simulink model "stanleyHighway"  (R2020b)
settings: Solver=VariableStepAuto  StartTime=0.0  StopTime=50  FixedStep=0.001  RelTol=1e-3
PreLoadFcn:
  | velocityProfile
  | setUpModel
  | close
model workspace (MAT data in the model file):
  firstWarning = 0
  originalScenarioChecksum = 'F73A6DA3C723D3CA73A6F931B7A52A9C'
undefined symbols (not defined in the file or in its folder): curvature, direction, dislt, distancecovered, gradbp, psi_o, q11, thetaRefab, velt_res, X_o, xRef2s, Y_o, yRef2s
libraries: vehdynlibtirecommon x4, autolibutils x4, simulink_extras x3, simulink x3, drivingvehiclecontroller x2, vehdynlibviscommon x1, drivingscenarioandsensors x1, vehdynlibtire x1, sim3dlib x1, vdynlib x1, autolibshared x1
settings Model: PacingRate=0.700000  Creator=valakshe  LastModifiedBy=valakshe

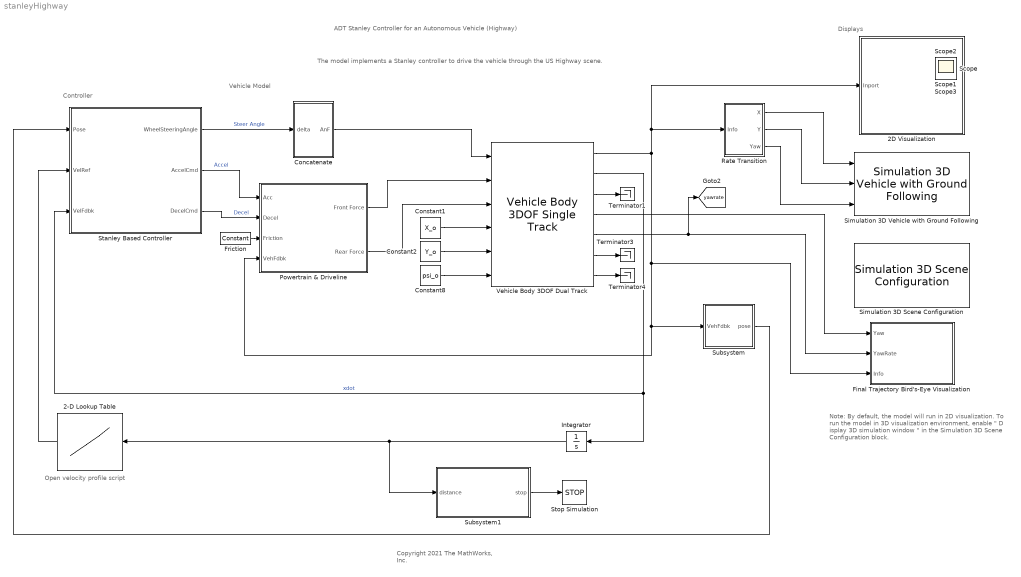
== system stanleyHighway ==
  note: Open velocity profile script
  note: Note: By default, the model will run in 2D visualization. To run the model in 3D visualization
      | environment, enable " D isplay 3D simulation window " in the Simulation 3D Scene Configuration block.
  note: Copyright 2021 The MathWorks, Inc.
  note: Controller
  note: Vehicle Model
  note: ADT Stanley Controller for an Autonomous Vehicle
      | (Highway)
  note: Displays
  note: The model implements a Stanley controller to drive the vehicle through the US Highway scene.
  2-D Lookup Table : Lookup_n-D  NumberOfTableDimensions=1  BreakpointsForDimension1=dislt;  BreakpointsForDimension2=q11(:,2)  Table=velt_res;  InterpMethod=Cubic spline  InternalRulePriority=Speed  RndMeth=Simplest  InputSameDT=on
  2D Visualization : Subsystem
      mask Display: image("visualization.JPG");
  Concatenate : Subsystem
  Constant1 : Constant  Value=X_o
  Constant2 : Constant  Value=Y_o
  Constant8 : Constant  Value=psi_o
  Final Trajectory Bird's-Eye Visualization : Subsystem
  Friction : vehdynlibtirecommon/Constant  const=1  numWheels=4
      settings: SourceProductBaseCode=VE
  Integrator : Integrator  InitialCondition=sqrt((X_o).^2+(Y_o).^2)
  Powertrain & Driveline : Subsystem
      mask Display: image('vdbslibpt.png');
  Rate Transition : Subsystem
  Simulation 3D Scene Configuration : sim3dlib/Simulation 3D Scene Configuration  Priority=1  ProjectFormat=Default Scenes  SceneDesc=US highway  ProjectName=C:\Fdrive\UnrealAutonomousVehicle\8MileUnrealexe\AutoVrtlEnv.exe  ScenePath=8mile  UEProjPath=C:\Local\AutoVrtlEnv\AutoVrtlEnv.uproject  vehTagList={'Scene Origin';'SimulinkVehicle1'}  vehTag=SimulinkVehicle1  OpVisEn=off  Ts=.05  EnableWindow=on  sensorTag=MainCamera1  sensorId=1  sensorName=MainCamera1  mountLoc=Origin  offsetFlag=off  tmountOffset=[0, 0, 0]  rmountOffset=[0, 0, 0]  HorizontalResolution=1280  VerticalResolution=720  HorizontalFOV=60  mountPoint=[0 0 0]  mountOrientation=[0 0 0]  aMode=2  ID=1
      settings: SourceProductBaseCode=DR,UV,VE
  Simulation 3D Vehicle with Ground Following : vdynlib/Vehicle Scenarios/Sim3D/Sim3D Vehicle/Components/Simulation 3D Vehicle with Ground Following  Priority=-1  PassVehMesh=Hatchback  VehColor=Green  InitialPos=[X_o,Y_o,-1]  InitialRot=[0, 0, psi_o]  ActorName=SimulinkVehicle1  SampleTime=-1  ActorType=SimulinkVehicle  ID=1  aMode=2  ActorTag=SimulinkVehicle1  CoordinateScheme=SAE
      settings: SourceProductBaseCode=VE
  Stanley Based Controller : Subsystem  VariantControl=Stanley
  Stop Simulation : Stop
  Subsystem : Subsystem
  Subsystem1 : Subsystem
  Terminator1 : Terminator
  Terminator3 : Terminator
  Terminator4 : Terminator
  Vehicle Body 3DOF Dual Track : autolibshared/Vehicle Body 3DOF Single Track  trackMode=Dual  inputMode=External forces  frontSteerMode=on  rearSteerMode=off  windMode=off  muMode=off  extFMode=off  extMMode=off  htchFMode=off  htchMMode=off  extXo=on  extpsio=on  extxdoto=off  extro=off  extYo=on  extTamb=off  extydoto=off  aMode=2  NF=2  NR=2  m=2000  a=1.4  b=1.6  h=0.35  dh=1  hh=0.2  X_o=0  xdot_o=velt_res(1)  CalphaMode=off  sigmaMode=on  d=0  hl=0  w=[1.4,1.4]  Cy_f=12e3  Cy_r=11e3  sigma_f=.1  sigma_r=.1  alpha_f_brk=[-.1 .1]  Cy_f_data=[-9e3 9e3]  alpha_r_brk=[-.1 .1]  Cy_r_data=[-9e3 9e3]  Y_o=0  ydot_o=0  Izz=4000  psi_o=0  r_o=0  Af=2  Cd=.3  Cl=.1  Cpm=.1  beta_w=[0:0.01:0.3]  Cs=[0:0.03:0.9]  Cym=[0:0.01:0.3]  Pabs=101325  Tair=273  g=9.81  mu=1  xdot_tol=.01  Fznom=5000  Fxtire_sat=7e4  Fytire_sat=7e4  longOff=0  latOff=0  vertOff=0  wrapAng=off
      settings: SourceProductBaseCode=PW,MT,UV,VE,VP
  Scope{,1..3} (4 alike) : Scope
  tag scope: yawrate=global
  wires:
  Vehicle Body 3DOF Dual Track/7 -> Terminator4/1
  Vehicle Body 3DOF Dual Track/4 -> Final Trajectory Bird's-Eye Visualization/1(Yaw)
  Powertrain & Driveline/1(Front Force) -> Vehicle Body 3DOF Dual Track/2
  Stanley Based Controller/3(DecelCmd) -> Powertrain & Driveline/2(Decel)  "Decel"
  Vehicle Body 3DOF Dual Track/1 -> Subsystem/1(VehFdbk), Powertrain & Driveline/4(VehFdbk), Final Trajectory Bird's-Eye Visualization/3(Info), Rate Transition/1(Info), 2D Visualization/1(Inport)
  Constant1/1 -> Vehicle Body 3DOF Dual Track/4
  Stanley Based Controller/1(WheelSteeringAngle) -> Concatenate/1(delta)  "Steer Angle"
  Vehicle Body 3DOF Dual Track/2 -> Integrator/1, Stanley Based Controller/3(VelFdbk)  "xdot"
  Vehicle Body 3DOF Dual Track/3 -> Terminator1/1
  Concatenate/1(AnF) -> Vehicle Body 3DOF Dual Track/1
  Vehicle Body 3DOF Dual Track/6 -> Terminator3/1
  Constant8/1 -> Vehicle Body 3DOF Dual Track/6
  Rate Transition/1(X) -> Simulation 3D Vehicle with Ground Following/1
  Powertrain & Driveline/2(Rear Force) -> Vehicle Body 3DOF Dual Track/3
  Vehicle Body 3DOF Dual Track/5 -> Final Trajectory Bird's-Eye Visualization/2(YawRate), [yawrate]
  Rate Transition/3(Yaw) -> Simulation 3D Vehicle with Ground Following/3
  Rate Transition/2(Y) -> Simulation 3D Vehicle with Ground Following/2
  Stanley Based Controller/2(AccelCmd) -> Powertrain & Driveline/1(Acc)  "Accel"
  Constant2/1 -> Vehicle Body 3DOF Dual Track/5
  Friction/1 -> Powertrain & Driveline/3(Friction)
  Subsystem/1(pose) -> Stanley Based Controller/1(Pose)
  Subsystem1/1(stop) -> Stop Simulation/1
  2-D Lookup Table/1 -> Stanley Based Controller/2(VelRef)
  Integrator/1 -> Subsystem1/1(distance), 2-D Lookup Table/1

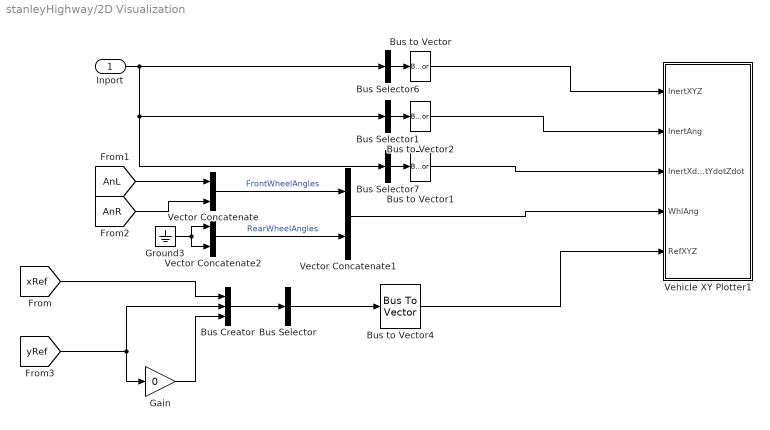
== system stanleyHighway/2D Visualization ==
  Inport : Inport
  Bus Creator : BusCreator  Inputs=3
  Bus Selector : BusSelector  OutputSignals=signal1,signal2,signal3  OutputAsBus=on
  Bus Selector1 : BusSelector  OutputSignals=InertFrm.Cg.Ang.phi,InertFrm.Cg.Ang.theta,InertFrm.Cg.Ang.psi  OutputAsBus=on
  Bus Selector6 : BusSelector  OutputSignals=InertFrm.Geom.Disp.X,InertFrm.Geom.Disp.Y,InertFrm.Geom.Disp.Z  OutputAsBus=on
  Bus Selector7 : BusSelector  OutputSignals=InertFrm.Geom.Vel.Xdot,InertFrm.Geom.Vel.Ydot,InertFrm.Geom.Vel.Zdot  OutputAsBus=on
  Bus to Vector{,1..2,4} (4 alike) : BusToVector
  Gain : Gain  Gain=0
  Ground3 : Ground
  Vector Concatenate : Concatenate
  Vector Concatenate1 : Concatenate
  Vector Concatenate2 : Concatenate
  Vehicle XY Plotter1 : Subsystem  mask(Vehicle XY Plotter){extRef=on, extStats=off, extTireF=off, a=2, b=2, w=2, figBorder=10, bufferSize=1024, velNorm=5, tireFNorm=1000, pltDT=0.2}
      mask prompts: extRef "Plot path reference, extRef"; extStats "Display speed, RPM and Gear"; extTireF "Display tire forces"; a "Distance to front axle from CG, a [m]:"; b "Distance to rear axle from CG, b [m]:"; w "Track width, w [m]:"; figBorder "Distance to figure borders, figBorder [m]:"; bufferSize "Path buffer sampe size, bufferSize []:"; velNorm "Velocity vector scaling, velNorm [m*s/m]:"; tireFNorm "Tire force vector scaling, tireFNorm [m/N]:"; pltDT "Plot update rate, pltDT [s]:"
      mask help:
      | This block will display a MATLAB figure which indicates the vehicle path, current position and heading velocity.
      | An optional path reference is also provided.
      mask init:
      | block = gcb;
      | if autoblkschecksimstopped(block)
      |     ParamNames = {'extRef';'extStats';'extTireF';'extTireF'};
      |     PortNames = {'RefXYZ';'Stats';'TireFx';'TireFy'};
      |     for idx=1:length(PortNames)
      |         InportOption  = {'built-in/Ground', [PortNames{idx}, ' Ground'];...
      |             'built-in/Inport',PortNames{idx}};
      |         if ~strcmp(get_param(block,ParamNames{idx}),'on')
      |             NewBlkHdl = autoblksreplaceblock(block, InportOption, 1);
      |             set_param(NewBlkHdl, 'ShowName', 'off');
      |         else
      |             autoblksreplaceblock(block, InportOption, 2);
      |         end
      |     end
      |     InportNames = {'InertXYZ';'InertAng';'InertXdotYdotZdot';'WhlAng';'RefXYZ';'Stats';'TireFx';'TireFy'};
      |     FoundNames = get_param(find_system(block, 'LookUnderMasks', 'all', 'SearchDepth', 1, 'FollowLinks', 'on', 'BlockType', 'Inport'), 'Name');
      |     [~,PortI] = intersect(InportNames, FoundNames);
      |     PortI = sort(PortI);
      |     for idx = 1:length(PortI)
      |         set_param([block, '/', InportNames{PortI(idx)}], 'Port', num2str(idx));
      |     end
      | end
      mask TypeOptions a: Vehicle XY Plotter/a
      mask TypeOptions b: Vehicle XY Plotter/b
      mask TypeOptions w: Vehicle XY Plotter/w
      mask TypeOptions figBorder: Vehicle XY Plotter/figBorder
      mask TypeOptions bufferSize: Vehicle XY Plotter/bufferSize
      mask TypeOptions velNorm: Vehicle XY Plotter/velNorm
      mask TypeOptions tireFNorm: Vehicle XY Plotter/tireFNorm
      mask DialogControl Container3 Prompt: Plot and Display Options
  wires:
  Vector Concatenate1/1 -> Vehicle XY Plotter1/4(WhlAng)
  Ground3/1 -> Vector Concatenate2/1, Vector Concatenate2/2
  Bus Selector6/1 -> Bus to Vector/1
  Vector Concatenate/1 -> Vector Concatenate1/1  "FrontWheelAngles"
  [AnL] -> Vector Concatenate/1
  Vector Concatenate2/1 -> Vector Concatenate1/2  "RearWheelAngles"
  Bus Selector7/1 -> Bus to Vector1/1
  Bus to Vector1/1 -> Vehicle XY Plotter1/3(InertXdotYdotZdot)
  Bus to Vector/1 -> Vehicle XY Plotter1/1(InertXYZ)
  Bus to Vector2/1 -> Vehicle XY Plotter1/2(InertAng)
  Bus Selector1/1 -> Bus to Vector2/1
  [AnR] -> Vector Concatenate/2
  Inport/1 -> Bus Selector7/1, Bus Selector1/1, Bus Selector6/1
  Bus to Vector4/1 -> Vehicle XY Plotter1/5(RefXYZ)
  Bus Selector/1 -> Bus to Vector4/1
  [yRef] -> Bus Creator/2, Gain/1
  Gain/1 -> Bus Creator/3
  [xRef] -> Bus Creator/1
  Bus Creator/1 -> Bus Selector/1

== system stanleyHighway/Concatenate ==
  delta : Inport
  Matrix Concatenate : Concatenate
  AnF : Outport  VectorParamsAs1DForOutWhenUnconnected=off
  tag scope: AnL=global, AnR=global
  wires:
  Matrix Concatenate/1 -> AnF/1
  delta/1 -> [AnL], [AnR], Matrix Concatenate/2, Matrix Concatenate/1

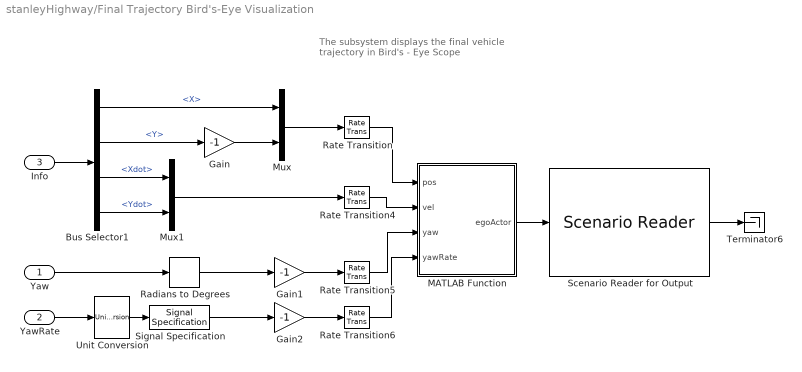
== system stanleyHighway/Final Trajectory Bird's-Eye Visualization ==
  note: The subsystem displays the final vehicle trajectory in Bird's - Eye Scope
  Yaw : Inport
  YawRate : Inport  Port=2
  Info : Inport  Port=3
  Bus Selector1 : BusSelector  OutputSignals=InertFrm.Cg.Disp.X,InertFrm.Cg.Disp.Y,InertFrm.Cg.Vel.Xdot,InertFrm.Cg.Vel.Ydot
  Gain : Gain  Gain=-1
  Gain1 : Gain  Gain=-1
  Gain2 : Gain  Gain=-1
  MATLAB Function : MATLAB Function  TreatAsAtomicUnit=on
  Mux : Mux  Inputs=2
  Mux1 : Mux  Inputs=2
  Radians to Degrees : simulink_extras/Transformations/Radians to Degrees
  Rate Transition{,4..6} (4 alike) : RateTransition
  "Scenario Reader for Output " : drivingscenarioandsensors/Scenario Reader  ScenarioSource=From file  ScenarioFileName=USHighway.mat  ScenarioVariableName=scenario  OutputCoordinateSystem=Vehicle coordinates  EgoVehicleSource=Input port  EgoVehicleActorID=1  OrientVehiclesOnRoad=off  OutputEgoVehiclePose=on  SampleTime=0.1  LaneBoundaryOutput=None  LaneBoundaryDistance=0:0.5:9.5  LaneBoundaryLocation=Center of lane markings  BusNameSource=Property  BusName=BusActors  BusName2Source=Auto  BusName2=BusLaneBoundaries  BusName3Source=Auto  BusName3=BusEgoActor  ShowCoordinateLabels=on  SimulateUsing=Interpreted execution
  Signal Specification : SignalSpecification  Unit=deg/s
  Terminator6 : Terminator
  Unit Conversion : UnitConversion
  wires:
  "Scenario Reader for Output "/1 -> Terminator6/1
  YawRate/1 -> Unit Conversion/1
  Yaw/1 -> Radians to Degrees/1
  Gain2/1 -> Rate Transition6/1
  Gain1/1 -> Rate Transition5/1
  Signal Specification/1 -> Gain2/1
  Radians to Degrees/1 -> Gain1/1
  Info/1 -> Bus Selector1/1
  Bus Selector1/3 -> Mux1/1  "<Xdot>"
  Mux/1 -> Rate Transition/1
  Gain/1 -> Mux/2
  Bus Selector1/4 -> Mux1/2  "<Ydot>"
  Rate Transition5/1 -> MATLAB Function/3(yaw)
  Mux1/1 -> Rate Transition4/1
  MATLAB Function/1(egoActor) -> "Scenario Reader for Output "/1
  Rate Transition4/1 -> MATLAB Function/2(vel)
  Bus Selector1/2 -> Gain/1  "<Y>"
  Bus Selector1/1 -> Mux/1  "<X>"
  Rate Transition/1 -> MATLAB Function/1(pos)
  Rate Transition6/1 -> MATLAB Function/4(yawRate)
  Unit Conversion/1 -> Signal Specification/1

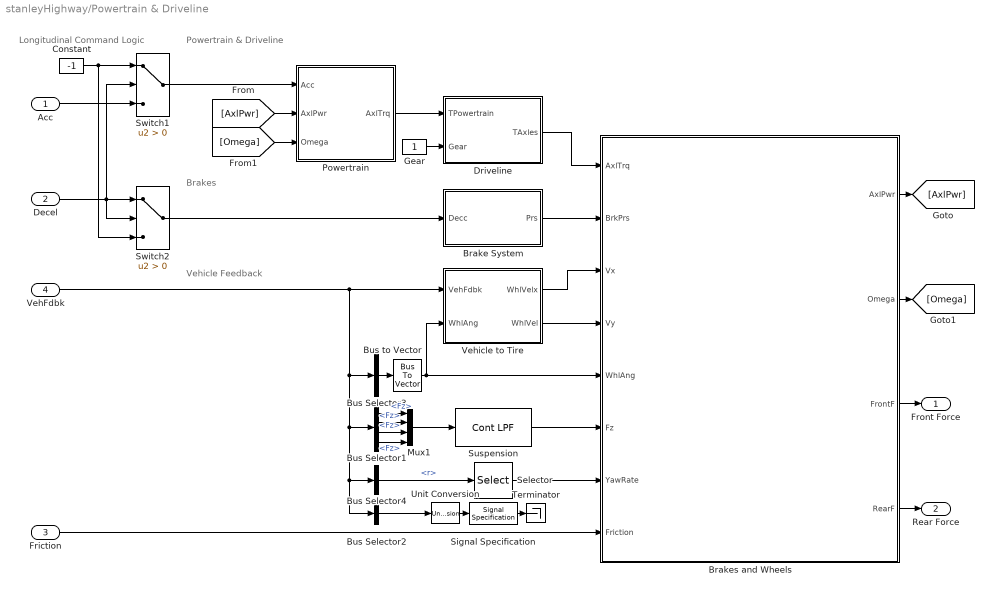
== system stanleyHighway/Powertrain & Driveline ==
  note: Vehicle Feedback
  note: Powertrain & Driveline
  note: Brakes
  note: Longitudinal Command Logic
  Acc : Inport
  Decel : Inport  Port=2
  Friction : Inport  Port=3
  VehFdbk : Inport  Port=4
  Brake System : Subsystem
  Brakes and Wheels : Subsystem  TreatAsAtomicUnit=on
      mask Display: image('vdbslibwhls.png');
  Bus Selector1 : BusSelector  OutputSignals=BdyFrm.Forces.Tires.FrntTires.Lft.Fz,BdyFrm.Forces.Tires.FrntTires.Rght.Fz,BdyFrm.Forces.Tires.RearTires.Lft.Fz,BdyFrm.Forces.Tires.RearTires.Rght.Fz
  Bus Selector2 : BusSelector  OutputSignals=BdyFrm.Cg.Vel.xdot  OutputAsBus=on
  Bus Selector3 : BusSelector  OutputSignals=BdyFrm.FrntAxl.Steer.WhlAngFL,BdyFrm.FrntAxl.Steer.WhlAngFR,BdyFrm.RearAxl.Steer.WhlAngRL,BdyFrm.RearAxl.Steer.WhlAngRR  OutputAsBus=on
  Bus Selector4 : BusSelector  OutputSignals=BdyFrm.Cg.AngVel.r
  Bus to Vector : BusToVector
  Constant : Constant  Value=-1
  Driveline : Subsystem  Variant=on  VariantControlMode=label  VariantControl=Variant1  LabelModeActiveChoice=0
  Gear : Constant
  Mux1 : Mux
  Powertrain : Subsystem
  Selector : Selector  InputPortWidth=1  IndexOptions=Index vector (dialog)  Indices=[1 1 1 1]  OutputSizes=1
  Signal Specification : SignalSpecification  Unit=km/hr
  Suspension : autolibutils/Cont LPF  wc=10*pi*2  aMode=2
      settings: SourceProductBaseCode=PW,MT,UV,VE,VP
  Switch1 : Switch  Criteria=u2 > Threshold
  Switch2 : Switch  Criteria=u2 > Threshold
  Terminator : Terminator
  Unit Conversion : UnitConversion
  Vehicle to Tire : Subsystem
  Front Force : Outport  VectorParamsAs1DForOutWhenUnconnected=off
  Rear Force : Outport  Port=2  VectorParamsAs1DForOutWhenUnconnected=off
  wires:
  Vehicle to Tire/2(WhlVel) -> Brakes and Wheels/4(Vy)
  Vehicle to Tire/1(WhlVelx) -> Brakes and Wheels/3(Vx)
  Brakes and Wheels/1(AxlPwr) -> [AxlPwr]
  Brakes and Wheels/4(RearF) -> Rear Force/1
  Brakes and Wheels/3(FrontF) -> Front Force/1
  Brakes and Wheels/2(Omega) -> [Omega]
  VehFdbk/1 -> Vehicle to Tire/1(VehFdbk), Bus Selector3/1, Bus Selector1/1, Bus Selector4/1, Bus Selector2/1
  Selector/1 -> Brakes and Wheels/7(YawRate)
  Bus Selector4/1 -> Selector/1  "<r>"
  Friction/1 -> Brakes and Wheels/8(Friction)
  Gear/1 -> Driveline/2(Gear)
  Signal Specification/1 -> Terminator/1
  Unit Conversion/1 -> Signal Specification/1
  Bus Selector2/1 -> Unit Conversion/1
  Brake System/1(Prs) -> Brakes and Wheels/2(BrkPrs)
  Switch2/1 -> Brake System/1(Decc)
  [Omega] -> Powertrain/3(Omega)
  [AxlPwr] -> Powertrain/2(AxlPwr)
  Powertrain/1(AxlTrq) -> Driveline/1(TPowertrain)
  Switch1/1 -> Powertrain/1(Acc)
  Bus Selector1/4 -> Mux1/4  "<Fz>"
  Bus Selector1/3 -> Mux1/3  "<Fz>"
  Bus Selector1/2 -> Mux1/2  "<Fz>"
  Bus Selector1/1 -> Mux1/1  "<Fz>"
  Suspension/1 -> Brakes and Wheels/6(Fz)
  Mux1/1 -> Suspension/1
  Bus to Vector/1 -> Brakes and Wheels/5(WhlAng), Vehicle to Tire/2(WhlAng)
  Bus Selector3/1 -> Bus to Vector/1
  Driveline/1(TAxles) -> Brakes and Wheels/1(AxlTrq)
  Constant/1 -> Switch1/1, Switch2/3
  Acc/1 -> Switch1/3
  Decel/1 -> Switch2/1, Switch2/2, Switch1/2

== system stanleyHighway/Rate Transition ==
  Info : Inport
  Bus Selector2 : BusSelector  OutputSignals=InertFrm.Geom.Disp.X,InertFrm.Geom.Disp.Y,InertFrm.Cg.Ang.psi
  Rate Transition1 : RateTransition  InitialCondition=X_o  OutPortSampleTime=0.01
  Rate Transition2 : RateTransition  InitialCondition=Y_o  OutPortSampleTime=0.01
  Rate Transition3 : RateTransition  OutPortSampleTime=0.01
  X : Outport
  Y : Outport  Port=2
  Yaw : Outport  Port=3
  wires:
  Info/1 -> Bus Selector2/1
  Rate Transition3/1 -> Yaw/1
  Rate Transition2/1 -> Y/1
  Rate Transition1/1 -> X/1
  Bus Selector2/1 -> Rate Transition1/1  "<X>"
  Bus Selector2/3 -> Rate Transition3/1  "<psi>"
  Bus Selector2/2 -> Rate Transition2/1  "<Y>"

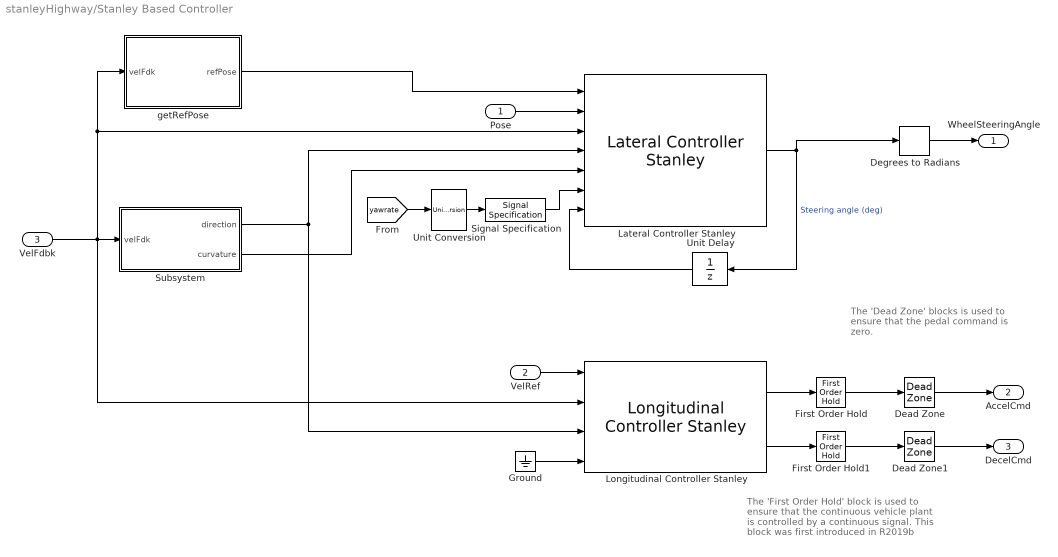
== system stanleyHighway/Stanley Based Controller ==
  note: The 'Dead Zone' blocks is used to ensure that the pedal command is zero.
  note: The 'First Order Hold' block is used to ensure that the continuous vehicle plant is controlled by a continuous signal. This block was first introduced in R2019b
  Pose : Inport
  VelRef : Inport  Port=2
  VelFdbk : Inport  Port=3
  Dead Zone : DeadZone  LowerValue=-0.001  UpperValue=0.001  SaturateOnIntegerOverflow=on
  Dead Zone1 : DeadZone  LowerValue=-0.001  UpperValue=0.001  SaturateOnIntegerOverflow=on
  Degrees to Radians : simulink_extras/Transformations/Degrees to Radians
  First Order Hold : FirstOrderHold  ErrorTolerance=inf
  First Order Hold1 : FirstOrderHold  ErrorTolerance=inf
  Ground : Ground
  Lateral Controller Stanley : drivingvehiclecontroller/Lateral Controller Stanley  ModelType=Dynamic bicycle model  PositionGainF=1  PositionGainR=1  YawRateGain=0.2  DelayGain=0.2  VehicleMass=2000  Lf=1.4  Lr=1.6  TireStiffness=12000  Wheelbase=3  MaxSteeringAngle=35
      settings: SourceProductBaseCode=DR
  Longitudinal Controller Stanley : drivingvehiclecontroller/Longitudinal Controller Stanley  Kp=0.6  Ki=0.5  SampleTime=0.05  MaxAcceleration=1  MaxDeceleration=1
      settings: SourceProductBaseCode=DR
  Signal Specification : SignalSpecification  Unit=deg/s
  Subsystem : Subsystem
  Unit Conversion : UnitConversion
  Unit Delay : UnitDelay  SampleTime=-1  HasFrameUpgradeWarning=on
  getRefPose : Subsystem
  WheelSteeringAngle : Outport
  AccelCmd : Outport  Port=2
  DecelCmd : Outport  Port=3
  wires:
  Longitudinal Controller Stanley/2 -> First Order Hold1/1
  VelFdbk/1 -> Longitudinal Controller Stanley/2, Subsystem/1(velFdk), getRefPose/1(velFdk), Lateral Controller Stanley/3
  Pose/1 -> Lateral Controller Stanley/2
  Ground/1 -> Longitudinal Controller Stanley/4
  Longitudinal Controller Stanley/1 -> First Order Hold/1
  Degrees to Radians/1 -> WheelSteeringAngle/1
  getRefPose/1(refPose) -> Lateral Controller Stanley/1
  [yawrate] -> Unit Conversion/1
  Signal Specification/1 -> Lateral Controller Stanley/6
  Lateral Controller Stanley/1 -> Degrees to Radians/1, Unit Delay/1  "Steering angle (deg)"
  Unit Delay/1 -> Lateral Controller Stanley/7
  Subsystem/1(direction) -> Longitudinal Controller Stanley/3, Lateral Controller Stanley/4
  VelRef/1 -> Longitudinal Controller Stanley/1
  Subsystem/2(curvature) -> Lateral Controller Stanley/5
  First Order Hold/1 -> Dead Zone/1
  First Order Hold1/1 -> Dead Zone1/1
  Dead Zone/1 -> AccelCmd/1
  Dead Zone1/1 -> DecelCmd/1
  Unit Conversion/1 -> Signal Specification/1

== system stanleyHighway/Subsystem ==
  VehFdbk : Inport
  Bus Selector : BusSelector  OutputSignals=InertFrm.Cg.Disp.X,InertFrm.Cg.Disp.Y,InertFrm.Cg.Ang.psi
  Gain1 : Gain  Gain=180/pi
  Mux : Mux  Inputs=3
  Transpose : Math  Operator=transpose  SignedPower=on  SaturateOnIntegerOverflow=on
  pose : Outport
  wires:
  Mux/1 -> Transpose/1
  VehFdbk/1 -> Bus Selector/1
  Bus Selector/1 -> Mux/1  "<X>"
  Gain1/1 -> Mux/3
  Bus Selector/2 -> Mux/2  "<Y>"
  Transpose/1 -> pose/1
  Bus Selector/3 -> Gain1/1  "<psi>"

== system stanleyHighway/Subsystem1 ==
  distance : Inport
  Constant : Constant
  Constant3 : Constant  Value=0
  Switch : Switch  Threshold=distancecovered-10
  stop : Outport
  wires:
  Switch/1 -> stop/1
  Constant3/1 -> Switch/3
  distance/1 -> Switch/2
  Constant/1 -> Switch/1

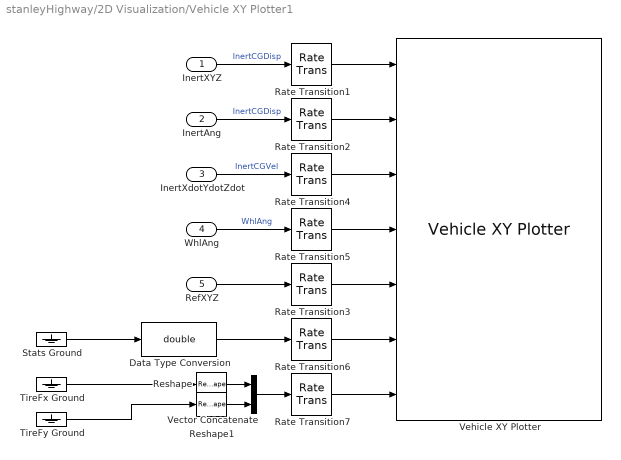
== system stanleyHighway/2D Visualization/Vehicle XY Plotter1 ==
  InertXYZ : Inport
  InertAng : Inport  Port=2
  InertXdotYdotZdot : Inport  Port=3
  WhlAng : Inport  Port=4
  RefXYZ : Inport  Port=5
  Data Type Conversion : DataTypeConversion  OutDataTypeStr=double
  Rate Transition{1..7} (7 alike) : RateTransition  Deterministic=off  OutPortSampleTime=pltDT
  Reshape : Reshape  OutputDimensionality=Row vector (2-D)
  Reshape1 : Reshape  OutputDimensionality=Row vector (2-D)
  Stats Ground : Ground
  TireFx Ground : Ground
  TireFy Ground : Ground
  Vector Concatenate : Concatenate  Mode=Multidimensional array
  Vehicle XY Plotter : vehdynlibviscommon/Vehicle XY Plotter  bufferSize=bufferSize  w=w  a=a  b=b  figBorder=figBorder  velNorm=velNorm  tireFNorm=tireFNorm
      settings: SourceProductBaseCode=VE
  wires:
  Vector Concatenate/1 -> Rate Transition7/1
  Reshape1/1 -> Vector Concatenate/2
  Reshape/1 -> Vector Concatenate/1
  RefXYZ/1 -> Rate Transition3/1
  Rate Transition7/1 -> Vehicle XY Plotter/7
  Data Type Conversion/1 -> Rate Transition6/1
  Rate Transition6/1 -> Vehicle XY Plotter/6
  Rate Transition5/1 -> Vehicle XY Plotter/4
  Rate Transition4/1 -> Vehicle XY Plotter/3
  Rate Transition2/1 -> Vehicle XY Plotter/2
  Rate Transition1/1 -> Vehicle XY Plotter/1
  Rate Transition3/1 -> Vehicle XY Plotter/5
  WhlAng/1 -> Rate Transition5/1  "WhlAng"
  InertXYZ/1 -> Rate Transition1/1  "InertCGDisp"
  InertXdotYdotZdot/1 -> Rate Transition4/1  "InertCGVel"
  InertAng/1 -> Rate Transition2/1  "InertCGDisp"
  Stats Ground/1 -> Data Type Conversion/1
  TireFx Ground/1 -> Reshape/1
  TireFy Ground/1 -> Reshape1/1

== system stanleyHighway/Powertrain & Driveline/Brake System ==
  Decc : Inport
  Hydraulics : autolibutils/Cont LPF  wc=30*pi*2  aMode=2
      settings: SourceProductBaseCode=PW,MT,UV,VE,VP
  Pressure : Gain  Gain=2e7
  Saturation1 : Saturate  UpperLimit=inf  LowerLimit=0  ZeroCross=off
  Selector : Selector  InputPortWidth=1  IndexOptions=Index vector (dialog)  Indices=[1 1 1 1]  OutputSizes=1
  Signal Specification : SignalSpecification  Unit=Pa
  Prs : Outport  PortDimensions=4  VectorParamsAs1DForOutWhenUnconnected=off
  wires:
  Signal Specification/1 -> Prs/1
  Decc/1 -> Saturation1/1
  Selector/1 -> Signal Specification/1
  Saturation1/1 -> Hydraulics/1
  Hydraulics/1 -> Pressure/1
  Pressure/1 -> Selector/1

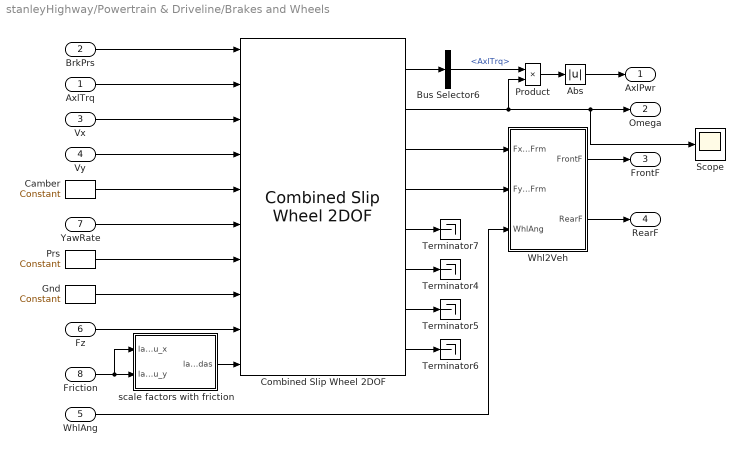
== system stanleyHighway/Powertrain & Driveline/Brakes and Wheels ==
  AxlTrq : Inport
  BrkPrs : Inport  Port=2
  Vx : Inport  Port=3
  Vy : Inport  Port=4
  WhlAng : Inport  Port=5
  Fz : Inport  Port=6  PortDimensions=4
  YawRate : Inport  Port=7
  Friction : Inport  Port=8
  Abs : Abs
  Bus Selector6 : BusSelector  OutputSignals=AxlTrq
  Camber : vehdynlibtirecommon/Constant  const=0  numWheels=4
      settings: SourceProductBaseCode=VE
  Combined Slip Wheel 2DOF : vehdynlibtire/Combined Slip Wheel 2DOF  BrakeType=Disc  mu_static=.3  mu_kinetic=.2  disk_abore=.05  Rm=.177  num_pads=2  drum_abore=0.0508  drum_a=0.123  drum_c=0.212  drum_r=0.15  drum_theta1=0  drum_theta2=126  brake_p_bpt=[1 11.4736842105263 21.9473684210526 32.4210526315789 42.8947368421053 53.3684210526316 63.8421052631579 74.3157894736842 84.7894736842105 95.2631578947368 105.736842105263 116.210526315789 126.684210526316 137.157894736842 147.631578947368 158.105263157895 168.578947368421 179.052631578947 189.526315789474 200]  brake_n_bpt=[0 52.6315789473684 105.263157894737 157.894736842105 210.526315789474 263.157894736842 315.789473684211 368.421052631579 421.052631578947 473.684210526316 526.315789473684 578.947368421053 631.578947368421 684.210526315789 736.842105263158 789.473684210526 842.105263157895 894.736842105263 947.368421052632 1000]  f_brake_t=[43.4900602404453 42.5056030554862 41.5350898940194 40.5780454442085 39.6340111501808 38.7025443887544 37.7832176914519 36.8756180088306 35.9793460143796 35.0940154454303 34.2192524787115 33.3546951383474 32.4999927342521 31.6548053290159 30.8188032315107 29.991666515561 29.1730845621415 28.362755623661 27.5603864089927 26.765691687993;498.991217495636 487.695866636631 476.560505099801 465.579679307235 454.748127933653 444.060772460445 433.51270824929 423.099196101319 412.81565427025 402.657650900201 392.620896861006 382.701238955775 372.894653477208 363.197240090814 353.605216024701 344.114910546964 334.722759712992 325.425301366216 316.219170376863 307.10109410434;954.492374750826 932.886130217776 911.585920305583 890.581313170261 869.862244717126 849.419000532136 829.242198807128 809.322774193808 789.651962526121 770.221286354971 751.0225412433 732.047782773203 713.289314220164 694.739674852612 676.391628817892 658.238154578366 640.272434863842 622.48784710877 604.877954344734 587.436496520688;1409.99353200602 1378.07639379892 1346.61133551136 1315.58294703329 1284.9763615006 1254.77722860383 1224.97168936497 1195.5463522863 1166.48827078199 1137.78492180974 1109.42418562559 1081.39432659063 1053.68397496312 1026.28210961441 999.178041611083 972.361398609768 945.822110014692 919.550392851325 893.536738312604 867.771898937035;1865.49468926121 1823.26665738007 1781.63675071715 1740.58458089631 1700.09047828407 1660.13545667552 1620.7011799228 1581.76993037878 1543.32457903786 1505.34855726451 1467.82583000789 1430.74087040806 1394.07863570608 1357.82454437621 1321.96445440427 1286.48464264117 1251.37178516554 1216.61293859388 1182.19552228048 1148.10730135338;2320.9958465164 2268.45692096121 2216.66216592293 2165.58621475934 2115.20459506754 2065.49368474721 2016.43067048064 1967.99350847127 1920.16088729373 1872.91219271928 1826.22747439018 1780.08741422549 1734.47329644903 1689.36697913801 1644.75086719747 1600.60788667257 1556.92146031639 1513.67548433643 1470.85430624835 1428.44270376973;2776.49700377159 2713.64718454235 2651.68758112871 2590.58784862237 2530.31871185102 2470.8519128189 2412.16016103848 2354.21708656376 2296.9971955496 2240.47582817405 2184.62911877248 2129.43395804292 2074.86795719199 2020.9094138998 1967.53727999066 1914.73113070398 1862.47113546724 1810.73803007899 1759.51309021622 1708.77810618608;3231.99816102678 3158.8374481235 3086.71299633449 3015.58948248539 2945.43282863449 2876.21014089059 2807.88965159632 2740.44066465625 2673.83350380547 2608.03946362882 2543.03076315477 2478.78050186034 2415.26261793494 2352.4518486616 2290.32369278385 2228.85437473538 2168.02081061809 2107.80057582154 2048.17187418409 1989.11350860242;3687.49931828197 3604.02771170464 3521.73841154027 3440.59111634842 3360.54694541796 3281.56836896228 3203.61914215416 3126.66424274874 3050.66981206134 2975.60309908359 2901.43240753707 2828.12704567777 2755.6572786779 2683.9942834234 2613.11010557704 2542.97761876678 2473.57048576894 2404.8631215641 2336.83065815196 2269.44891101877;4143.00047553716 4049.21797528579 3956.76382674606 3865.59275021144 3775.66106220143 3686.92659703397 3599.34863271199 3512.88782084123 3427.50612031721 3343.16673453836 3259.83405191936 3177.4735894952 3096.05193942085 3015.5367181852 2935.89651837023 2857.10086279818 2779.12016091979 2701.92566730665 2625.48944211983 2549.78431343512;4598.50163279235 4494.40823886693 4391.78924195184 4290.59438407447 4190.77517898491 4092.28482510566 3995.07812326983 3899.11139893372 3804.34242857308 3710.73036999313 3618.23569630166 3526.82013331263 3436.44660016381 3347.079152947 3258.68293116342 3171.22410682959 3084.66983607064 2998.98821304921 2914.1482260877 2830.11971585147;5054.00279004754 4939.59850244808 4826.81465715762 4715.59601793749 4605.88929576838 4497.64305317735 4390.80761382767 4285.3349770262 4181.17873682896 4078.2940054479 3976.63734068395 3876.16667713006 3776.84126090677 3678.62158770879 3581.46934395661 3485.34735086099 ...(+2764 chars)]  tireParamSet=vdynPassCar.mat  plySteer=off  turnslip=off  PRESMAX=1003118  PRESMIN=9982  FZMAX=10000  FZMIN=100  VXLOW=.01  KPUMAX=1  KPUMIN=-1  ALPMAX=pi/2  ALPMIN=-pi/2  CAMMAX=0.173142086627737  CAMMIN=-0.173348165334087  LONGVL=16.7  omegao=10/.309  br=1e-3  UNLOADED_RADIUS=0.309  NOMPRES=224006  FNOMIN=4025  WIDTH=0.209  RIM_RADIUS=.19  MASS=9.465  IYY=0.7406  GRAVITY=-9.81  zo=0  zdoto=0  BREFF=8.25094594147963  DREFF=0.260468730454265  FREFF=0.0735298544471851  Q_RE0=1.00866439868088  Q_V1=0.000760413786224011  Q_V2=0.0463384792019201  Q_FZ1=0  Q_FZ2=15.6870832810226  Q_FZ3=0  Q_FCX=0.138643970247602  Q_FCY=0.10843499565426  Q_FCY2=-0.465763352339538  PFZ1=0.69958166705601  VERTICAL_STIFFNESS=207885.061134007  VERTICAL_DAMPING=494.649255786991  BOTTOM_OFFST=.01  BOTTOM_STIFF=2e6  LONGITUDINAL_STIFFNESS=388714.175879854  LATERAL_STIFFNESS=157087.404633332  PCFX1=0.18539229191199  PCFX2=0  PCFX3=0  PCFY1=0.163183345037677  PCFY2=0  PCFY3=0.249094918231954  Q_RA1=0.675942571700787  Q_RA2=0.73800463546164  Q_RB1=1.04487486456705  Q_RB2=-1.191763806629  PCX1=1.58523057950359  PDX1=1.0239116238178  PDX2=-0.0842405110022724  PDX3=0  PEX1=0.110312777158455  PEX2=0.313468516038146  PEX3=0  PEX4=0.0016060905760045  PKX1=21.3872544684023  PKX2=14.0006541873175  PKX3=-0.405326109653452  PHX1=0.000212599305364818  PHX2=0.00115950515263055  PVX1=1.59236164471432e-05  PVX2=0.000104321112127671  PPX1=-0.349461321276586  PPX2=0.387840040616429  PPX3=-0.0969947336569324  PPX4=0.0632271859795801  RBX1=12.7633329850276  RBX2=9.5787123658471  RBX3=0  RCX1=1.02796280922059  REX1=-0.45202516851367  REX2=-0.47304886171176  RHX1=0.000233272373115809  QSX1=-0.00788307788961443  QSX2=0.954629515459396  QSX3=0.0155855777667025  QSX4=0.125904607142414  QSX5=1.01110069703963  QSX6=20.1938577118433  QSX7=0.310818120717083  QSX8=-0.0430823751139655  QSX9=0.636494404888216  QSX10=0.142438060591663  QSX11=0.346766530036373  QSX12=0  QSX13=0  QSX14=0  PPMX1=0  PCY1=1.34299950037631  PDY1=0.878267729082195  PDY2=-0.0644597923147385  PDY3=0  PEY1=-0.809776534470972  PEY2=-0.600180598867198  PEY3=0.0991732552633487  PEY4=-6.5577974035573  PEY5=0  PKY1=-15.5714726518315  PKY2=1.73126522291751  PKY3=0.365349873517229  PKY4=1.98176755955416  PKY5=0  PKY6=-0.884005199550313  PKY7=-0.237259727611847  PHY1=-0.00183370557235628  PHY2=0.00346401302716671  PVY1=-0.00675427560163264  PVY2=0.036379218103843  PVY3=-0.163543984089166  PVY4=-0.491003349625726  PPY1=-0.62059646553185  PPY2=-0.0647824842338686  PPY3=-0.164648843290686  PPY4=0.283193909060098  PPY5=0  RBY1=10.7588809173639  RBY2=7.70420065295029  RBY3=3.40283755070691e-06  RBY4=0  RCY1=1.06691874059059  REY1=0.308244924574305  REY2=7.48775032604508e-06  RHY1=0.0118479204960415  RHY2=7.63650177161071e-06  RVY1=0.0560024425050078  RVY2=7.48487127056197e-06  RVY3=0  RVY4=98.4047026517149  RVY5=2.02759273900054  RVY6=15.7623064923347  QSY1=0.00699077564863536  QSY2=0  QSY3=0.00153535478298811  QSY4=8.55710322455322e-05  QSY5=0  QSY6=0  QSY7=0.89443879773793  QSY8=-0.403227641260894  QBZ1=11.666656027484  QBZ2=-1.30355438574485  QBZ3=0  QBZ4=0.177918305399071  QBZ5=-0.162481135068033  QBZ6=0  QBZ9=30.1445534682089  QBZ10=0  QCZ1=1.29026978207574  QDZ1=0.0886972644991399  QDZ2=-0.0058634820161856  QDZ3=0.3805597481383  QDZ4=0  QDZ6=0.00160914918118959  QDZ7=-0.00211036330862154  QDZ8=-0.13921904912557  QDZ9=0.00816585550028243  QDZ10=0  QDZ11=0  QEZ1=-2.19802254534746  QEZ2=1.01850535789165  QEZ3=0  QEZ4=0.278379679112054  QEZ5=-0.548414722765386  QHZ1=0.00148361198869669  QHZ2=0.00202017567585904  QHZ3=0.240316641332066  QHZ4=-0.210114035738085  PPZ1=-0.443927982388615  PPZ2=0  SSZ1=0.00914999585397887  SSZ2=0.0389830656052735  SSZ3=0  SSZ4=0  PDXP1=0.396718274678791  PDXP2=0  PDXP3=0  PKYP1=1.00587060633573  PDYP1=0.40483048923438  PDYP2=0  PDYP3=0  PDYP4=0  PHYP1=0.992731942067188  PHYP2=0.150352945499914  PHYP3=0  PHYP4=-3.98988682633674  PECP1=0.502379254513503  PECP2=0  QDTP1=10.0178654287947  QCRP1=0.200627747200702  QCRP2=0.0995735881599772  QBRP1=0.0997107127960717  QDRP1=1.01432910167423  QDRP2=0  aMode=2
      settings: SourceProductBaseCode=VE
  Gnd : vehdynlibtirecommon/Constant  const=0  numWheels=4
      settings: SourceProductBaseCode=VE
  Product : Product
  Prs : vehdynlibtirecommon/Constant  const=2.4e5  numWheels=4
      settings: SourceProductBaseCode=VE
  Scope : Scope
  Terminator{4..7} (4 alike) : Terminator
  Whl2Veh : Subsystem
  scale factors with friction : Subsystem  mask{numWheels=4}
      mask prompts: numWheels "Number of wheels"
  AxlPwr : Outport
  Omega : Outport  Port=2
  FrontF : Outport  Port=3
  RearF : Outport  Port=4
  wires:
  scale factors with friction/1(lambdas) -> Combined Slip Wheel 2DOF/10
  Whl2Veh/2(RearF) -> RearF/1
  Whl2Veh/1(FrontF) -> FrontF/1
  Bus Selector6/1 -> Product/1  "<AxlTrq>"
  Abs/1 -> AxlPwr/1
  Combined Slip Wheel 2DOF/4 -> Whl2Veh/2(FyWhlFrm)
  Friction/1 -> scale factors with friction/2(lamda_mu_y), scale factors with friction/1(lamda_mu_x)
  Prs/1 -> Combined Slip Wheel 2DOF/7
  Combined Slip Wheel 2DOF/8 -> Terminator6/1
  Combined Slip Wheel 2DOF/5 -> Terminator7/1
  YawRate/1 -> Combined Slip Wheel 2DOF/6
  Combined Slip Wheel 2DOF/3 -> Whl2Veh/1(FxWhlFrm)
  AxlTrq/1 -> Combined Slip Wheel 2DOF/2
  Vy/1 -> Combined Slip Wheel 2DOF/4
  Vx/1 -> Combined Slip Wheel 2DOF/3
  Fz/1 -> Combined Slip Wheel 2DOF/9
  WhlAng/1 -> Whl2Veh/3(WhlAng)
  Product/1 -> Abs/1
  BrkPrs/1 -> Combined Slip Wheel 2DOF/1
  Combined Slip Wheel 2DOF/6 -> Terminator4/1
  Camber/1 -> Combined Slip Wheel 2DOF/5
  Combined Slip Wheel 2DOF/7 -> Terminator5/1
  Combined Slip Wheel 2DOF/2 -> Product/2, Scope/1, Omega/1
  Combined Slip Wheel 2DOF/1 -> Bus Selector6/1
  Gnd/1 -> Combined Slip Wheel 2DOF/8

== system stanleyHighway/Powertrain & Driveline/Driveline ==
  TPowertrain : Inport  PortDimensions=1
  Gear : Inport  Port=2
  AWD : Subsystem  VariantControl=2
  FWD : Subsystem  VariantControl=1
  RWD : Subsystem  VariantControl=0
  TAxles : Outport  PortDimensions=4  VectorParamsAs1DForOutWhenUnconnected=off

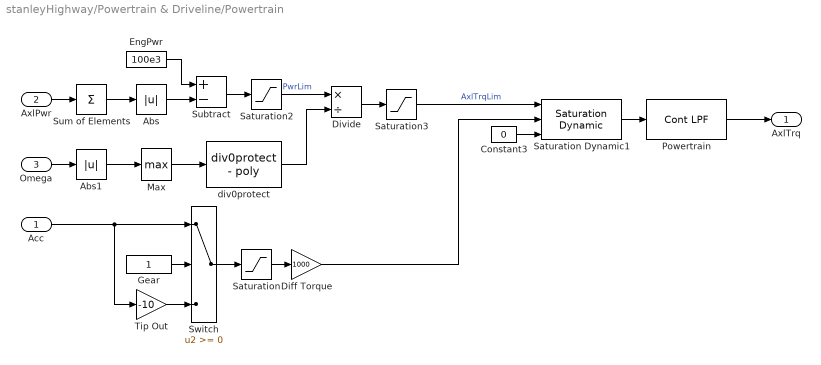
== system stanleyHighway/Powertrain & Driveline/Powertrain ==
  Acc : Inport
  AxlPwr : Inport  Port=2  PortDimensions=4
  Omega : Inport  Port=3  PortDimensions=4
  Abs : Abs  ZeroCross=off
  Abs1 : Abs  ZeroCross=off
  Constant3 : Constant  Value=0
  Diff Torque : Gain  Gain=1000
  Divide : Product  Inputs=*/
  EngPwr : Constant  Value=100e3
  Gear : Constant  SampleTime=-1
  Max : MinMax  Function=max  ZeroCross=off
  Powertrain : autolibutils/Cont LPF  wc=4*pi*2  aMode=2
      settings: SourceProductBaseCode=PW,MT,UV,VE,VP
  Saturation : Saturate  UpperLimit=inf  LowerLimit=0  ZeroCross=off
  Saturation Dynamic1 : simulink/Discontinuities/Saturation Dynamic  OutMin=[]  OutMax=[]  OutDataTypeStr=Inherit: Same as second input  OutDataType=fixdt(1, 16)  OutScaling=2^-10  DoSatur=off
  Saturation2 : Saturate  UpperLimit=inf  LowerLimit=100  ZeroCross=off
  Saturation3 : Saturate  UpperLimit=1000  LowerLimit=0  ZeroCross=off
  Subtract : Sum  Inputs=+-
  Sum of Elements : Sum  Inputs=+
  Switch : Switch  ZeroCross=off
  Tip Out : Gain  Gain=-10
  div0protect : autolibutils/div0protect - poly  thresh=1  aMode=2
      settings: SourceProductBaseCode=PW,MT,UV,VE,VP
  AxlTrq : Outport  VectorParamsAs1DForOutWhenUnconnected=off
  wires:
  Abs1/1 -> Max/1
  Max/1 -> div0protect/1
  Saturation3/1 -> Saturation Dynamic1/1  "AxlTrqLim"
  AxlPwr/1 -> Sum of Elements/1
  EngPwr/1 -> Subtract/1
  Saturation2/1 -> Divide/1  "PwrLim"
  Subtract/1 -> Saturation2/1
  Omega/1 -> Abs1/1
  div0protect/1 -> Divide/2
  Divide/1 -> Saturation3/1
  Abs/1 -> Subtract/2
  Sum of Elements/1 -> Abs/1
  Constant3/1 -> Saturation Dynamic1/3
  Tip Out/1 -> Switch/3
  Saturation Dynamic1/1 -> Powertrain/1
  Gear/1 -> Switch/2
  Diff Torque/1 -> Saturation Dynamic1/2
  Saturation/1 -> Diff Torque/1
  Acc/1 -> Switch/1, Tip Out/1
  Switch/1 -> Saturation/1
  Powertrain/1 -> AxlTrq/1

== system stanleyHighway/Powertrain & Driveline/Vehicle to Tire ==
  VehFdbk : Inport
  WhlAng : Inport  Port=2
  Bus Selector : BusSelector  OutputSignals=BdyFrm.FrntAxl.Lft.Vel.xdot,BdyFrm.FrntAxl.Rght.Vel.xdot,BdyFrm.RearAxl.Lft.Vel.xdot,BdyFrm.RearAxl.Rght.Vel.xdot,BdyFrm.FrntAxl.Lft.Vel.ydot,BdyFrm.FrntAxl.Rght.Vel.ydot,BdyFrm.RearAxl.Lft.Vel.ydot,BdyFrm.RearAxl.Rght.Vel.ydot
  Mux : Mux
  Mux2 : Mux
  Veh2Whl : Subsystem
  WhlVelx : Outport
  WhlVel : Outport  Port=2
  wires:
  WhlAng/1 -> Veh2Whl/3(WhlAng)
  Veh2Whl/2(VyWhlFrm) -> WhlVel/1
  Veh2Whl/1(VxWhlFrm) -> WhlVelx/1
  Mux2/1 -> Veh2Whl/2(Vy)
  Mux/1 -> Veh2Whl/1(Vx)
  VehFdbk/1 -> Bus Selector/1
  Bus Selector/1 -> Mux/1  "<xdot>"
  Bus Selector/7 -> Mux2/3  "<ydot>"
  Bus Selector/8 -> Mux2/4  "<ydot>"
  Bus Selector/6 -> Mux2/2  "<ydot>"
  Bus Selector/4 -> Mux/4  "<xdot>"
  Bus Selector/2 -> Mux/2  "<xdot>"
  Bus Selector/3 -> Mux/3  "<xdot>"
  Bus Selector/5 -> Mux2/1  "<ydot>"

== system stanleyHighway/Stanley Based Controller/Subsystem ==
  velFdk : Inport
  Curvature : Lookup_n-D  NumberOfTableDimensions=1  BreakpointsForDimension1=gradbp  Table=curvature  InternalRulePriority=Speed  RndMeth=Simplest  InputSameDT=on
  Direction : Lookup_n-D  NumberOfTableDimensions=1  BreakpointsForDimension1=gradbp  Table=direction  InternalRulePriority=Speed  RndMeth=Simplest  InputSameDT=on
  Integrator1 : Integrator
  direction : Outport
  curvature : Outport  Port=2
  wires:
  velFdk/1 -> Integrator1/1
  Integrator1/1 -> Direction/1, Curvature/1
  Curvature/1 -> curvature/1
  Direction/1 -> direction/1

== system stanleyHighway/Stanley Based Controller/getRefPose ==
  note: Select method to calculate theta
  velFdk : Inport
  Integrator : Integrator
  Mux : Mux  Inputs=3
  Theta : Subsystem  Variant=on  VariantControlMode=label  LabelModeActiveChoice=thetaSimulinkBlock
  X Ref : Lookup_n-D  NumberOfTableDimensions=1  BreakpointsForDimension1=gradbp  Table=xRef2s  InternalRulePriority=Speed  RndMeth=Simplest  InputSameDT=on
  Y Ref : Lookup_n-D  NumberOfTableDimensions=1  BreakpointsForDimension1=gradbp  Table=yRef2s  InternalRulePriority=Speed  RndMeth=Simplest  InputSameDT=on
  refPose : Outport
  tag scope: xRef=global, yRef=global
  wires:
  Integrator/1 -> X Ref/1, Theta/3(dis), Y Ref/1
  velFdk/1 -> Integrator/1
  Mux/1 -> refPose/1
  X Ref/1 -> Theta/2(x), [xRef], Mux/1
  Y Ref/1 -> Theta/1(y), [yRef], Mux/2
  Theta/1(theta) -> Mux/3

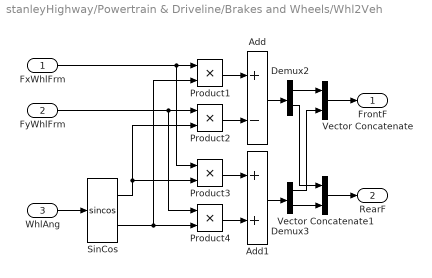
== system stanleyHighway/Powertrain & Driveline/Brakes and Wheels/Whl2Veh ==
  FxWhlFrm : Inport  PortDimensions=4
  FyWhlFrm : Inport  Port=2  PortDimensions=4
  WhlAng : Inport  Port=3
  Add : Sum  Inputs=+-
  Add1 : Sum
  Demux2 : Demux  Outputs=[2 2]
  Demux3 : Demux  Outputs=[2 2]
  Product{1..4} (4 alike) : Product
  SinCos : Trigonometry  Operator=sincos
  Vector Concatenate : Concatenate  Mode=Multidimensional array  ConcatenateDimension=2
  Vector Concatenate1 : Concatenate  Mode=Multidimensional array  ConcatenateDimension=2
  FrontF : Outport
  RearF : Outport  Port=2
  wires:
  Vector Concatenate/1 -> FrontF/1
  Demux3/1 -> Vector Concatenate/2
  Demux2/1 -> Vector Concatenate/1
  Demux2/2 -> Vector Concatenate1/1
  Demux3/2 -> Vector Concatenate1/2
  Vector Concatenate1/1 -> RearF/1
  Product4/1 -> Add1/2
  Add/1 -> Demux2/1
  Product2/1 -> Add/2
  SinCos/1 -> Product2/2, Product3/2
  Product1/1 -> Add/1
  SinCos/2 -> Product4/2, Product1/2
  FyWhlFrm/1 -> Product4/1, Product2/1
  Add1/1 -> Demux3/1
  FxWhlFrm/1 -> Product3/1, Product1/1
  Product3/1 -> Add1/1
  WhlAng/1 -> SinCos/1

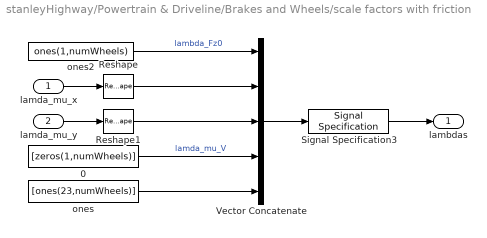
== system stanleyHighway/Powertrain & Driveline/Brakes and Wheels/scale factors with friction ==
  lamda_mu_x : Inport
  lamda_mu_y : Inport  Port=2
  0 : Constant  Value=[zeros(1,numWheels)]  VectorParams1D=off
  Reshape : Reshape  OutputDimensionality=Row vector (2-D)  OutputDimensions=[1,numWheels]
  Reshape1 : Reshape  OutputDimensionality=Row vector (2-D)  OutputDimensions=[1,numWheels]
  Signal Specification3 : SignalSpecification  Unit=1
  Vector Concatenate : Concatenate  NumInputs=5  Mode=Multidimensional array
  ones : Constant  Value=[ones(23,numWheels)]  VectorParams1D=off
  ones2 : Constant  Value=ones(1,numWheels)  VectorParams1D=off
  lambdas : Outport  Unit=1  VectorParamsAs1DForOutWhenUnconnected=off
  wires:
  Signal Specification3/1 -> lambdas/1
  Reshape/1 -> Vector Concatenate/2
  Reshape1/1 -> Vector Concatenate/3
  0/1 -> Vector Concatenate/4  "lamda_mu_V"
  ones/1 -> Vector Concatenate/5
  Vector Concatenate/1 -> Signal Specification3/1
  ones2/1 -> Vector Concatenate/1  "lambda_Fz0"
  lamda_mu_x/1 -> Reshape/1
  lamda_mu_y/1 -> Reshape1/1

== system stanleyHighway/Powertrain & Driveline/Driveline/AWD ==
  TPowertrain : Inport
  Gear : Inport  Port=2
  AWD : Gain  Gain=[1;1;1;1]./2
  Add : Sum
  Constant : Constant
  Constant1 : Constant  Value=zeros(4,1)
  Multiport Switch : MultiPortSwitch  DataPortOrder=Zero-based contiguous  zeroidx=on
  Unary Minus : UnaryMinus
  TAxles : Outport  VectorParamsAs1DForOutWhenUnconnected=off
  wires:
  Unary Minus/1 -> Multiport Switch/2
  Gear/1 -> Add/1
  Constant/1 -> Add/2
  AWD/1 -> Multiport Switch/4, Unary Minus/1
  Constant1/1 -> Multiport Switch/3
  Add/1 -> Multiport Switch/1
  Multiport Switch/1 -> TAxles/1
  TPowertrain/1 -> AWD/1

== system stanleyHighway/Powertrain & Driveline/Driveline/FWD ==
  TPowertrain : Inport
  Gear : Inport  Port=2
  Add : Sum
  Constant : Constant
  Constant1 : Constant  Value=zeros(4,1)
  FWD : Gain  Gain=[1;1;0;0]
  Multiport Switch : MultiPortSwitch  DataPortOrder=Zero-based contiguous  zeroidx=on
  Unary Minus : UnaryMinus
  TAxles : Outport  VectorParamsAs1DForOutWhenUnconnected=off
  wires:
  Unary Minus/1 -> Multiport Switch/2
  Gear/1 -> Add/1
  Constant/1 -> Add/2
  FWD/1 -> Multiport Switch/4, Unary Minus/1
  Constant1/1 -> Multiport Switch/3
  Add/1 -> Multiport Switch/1
  Multiport Switch/1 -> TAxles/1
  TPowertrain/1 -> FWD/1

== system stanleyHighway/Powertrain & Driveline/Driveline/RWD ==
  TPowertrain : Inport
  Gear : Inport  Port=2
  Add : Sum
  Constant : Constant
  Constant1 : Constant  Value=zeros(4,1)
  Multiport Switch : MultiPortSwitch  DataPortOrder=Zero-based contiguous  zeroidx=on
  RWD : Gain  Gain=[0;0;1;1]
  Unary Minus : UnaryMinus
  TAxles : Outport  VectorParamsAs1DForOutWhenUnconnected=off
  wires:
  Constant1/1 -> Multiport Switch/3
  Add/1 -> Multiport Switch/1
  Constant/1 -> Add/2
  Gear/1 -> Add/1
  Multiport Switch/1 -> TAxles/1
  Unary Minus/1 -> Multiport Switch/2
  TPowertrain/1 -> RWD/1
  RWD/1 -> Multiport Switch/4, Unary Minus/1

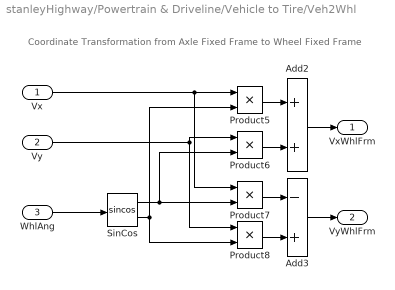
== system stanleyHighway/Powertrain & Driveline/Vehicle to Tire/Veh2Whl ==
  note: Coordinate Transformation from Axle Fixed Frame to Wheel Fixed Frame
  Vx : Inport
  Vy : Inport  Port=2
  WhlAng : Inport  Port=3
  Add2 : Sum
  Add3 : Sum  Inputs=-+
  Product{5..8} (4 alike) : Product
  SinCos : Trigonometry  Operator=sincos
  VxWhlFrm : Outport
  VyWhlFrm : Outport  Port=2
  wires:
  Add2/1 -> VxWhlFrm/1
  Add3/1 -> VyWhlFrm/1
  Product7/1 -> Add3/1
  Vy/1 -> Product8/1, Product6/1
  SinCos/2 -> Product8/2, Product5/2
  SinCos/1 -> Product7/2, Product6/2
  Product5/1 -> Add2/1
  Product6/1 -> Add2/2
  Product8/1 -> Add3/2
  Vx/1 -> Product5/1, Product7/1
  WhlAng/1 -> SinCos/1

== system stanleyHighway/Stanley Based Controller/getRefPose/Theta ==
  note: 1) Add Subsystem or Model blocks as valid variant choices.
      | 2) You cannot connect blocks at this level. At simulation, connectivity is automatically
      | determined, based on the active variant and port name matching.
  y : Inport
  x : Inport  Port=2
  dis : Inport  Port=3
  thetaBlocks : Subsystem  VariantControl=thetaSimulinkBlock
  thetaLt : Subsystem  VariantControl=thetaLookUpTable
  theta : Outport

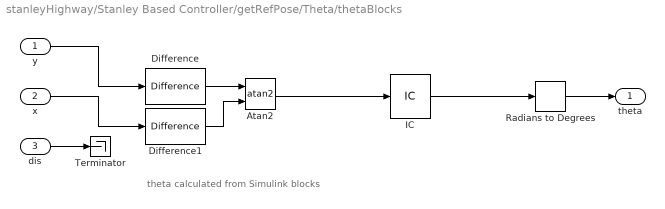
== system stanleyHighway/Stanley Based Controller/getRefPose/Theta/thetaBlocks ==
  note: theta calculated from Simulink blocks
  y : Inport
  x : Inport  Port=2
  dis : Inport  Port=3
  Atan2 : Trigonometry  Operator=atan2
  Difference : simulink/Discrete/Difference  ICPrevInput=0.0  OutMin=[]  OutMax=[]  OutDataType=fixdt(1, 16)  OutScaling=2^-10  DoSatur=off
  Difference1 : simulink/Discrete/Difference  ICPrevInput=0.0  OutMin=[]  OutMax=[]  OutDataType=fixdt(1, 16)  OutScaling=2^-10  DoSatur=off
  IC : InitialCondition  Value=psi_o
  Radians to Degrees : simulink_extras/Transformations/Radians to Degrees
  Terminator : Terminator
  theta : Outport
  wires:
  IC/1 -> Radians to Degrees/1
  Atan2/1 -> IC/1
  dis/1 -> Terminator/1
  x/1 -> Difference1/1
  y/1 -> Difference/1
  Radians to Degrees/1 -> theta/1
  Difference/1 -> Atan2/1
  Difference1/1 -> Atan2/2

== system stanleyHighway/Stanley Based Controller/getRefPose/Theta/thetaLt ==
  note: Check out the script "setUpModel" to understand how we have calculated theta
  note: theta based on lookup table
  y : Inport
  x : Inport  Port=2
  dis : Inport  Port=3
  Terminator : Terminator
  Terminator1 : Terminator
  Theta Ref : Lookup_n-D  NumberOfTableDimensions=1  BreakpointsForDimension1=gradbp  Table=thetaRefab  InternalRulePriority=Speed  RndMeth=Simplest  InputSameDT=on
  theta : Outport
  wires:
  Theta Ref/1 -> theta/1
  dis/1 -> Theta Ref/1
  x/1 -> Terminator1/1
  y/1 -> Terminator/1

== matlab function stanleyHighway/Final Trajectory Bird's-Eye Visualization/MATLAB Function ==
  data: pos input; egoActor output Bus: BusActorsActors; vel input; yaw input; yawRate input
function egoActor = packEgo(pos,vel,yaw,yawRate)
% Pack ego information into a single ego actor bus
%
% Imoprtant note:
% Output is a bus of type BusActorsActors. This is the same bus used by the
% Scenario Reader to output an individual actor. If you change the
% output bus name of Scenario Reader, change the output bus name here
% as well by clicking on 'Edit Data' in the menu above.

egoActor = struct(...
    'ActorID',46,...
    'Position', [pos(1) pos(2) 0], ...
    'Velocity', [vel(1) vel(2) 0], ...
    'Roll', 0, ...
    'Pitch', 0, ...
    'Yaw', yaw, ...
    'AngularVelocity', [0 0 yawRate]);
